simulink model "fixed_time_MASs"  (R2023b)
settings: Solver=FixedStepAuto  StartTime=0.0  StopTime=20  FixedStep=0.0001  RelTol=1e-3
(part 1 of 2)
settings Model: Creator=hxk  LastModifiedBy=hxk

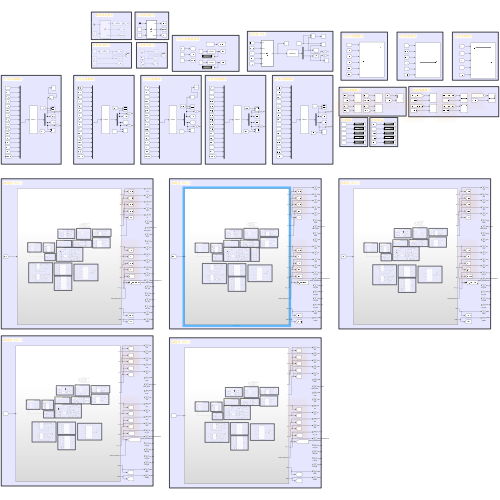
[thumbnail: Simulink's stored preview of the top-level diagram]
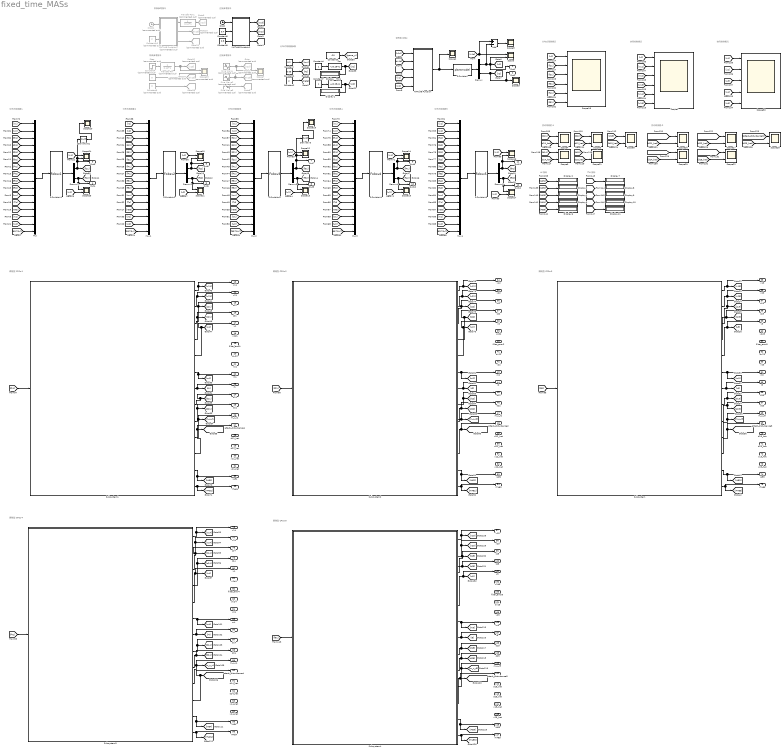
== system fixed_time_MASs ==
  note: 分布式观测情况
  note: 分布式观测器3
  note: 领导型 CPSs
  note: 分布式观测器1
  note: 分布式观测器2
  note: 分布式观测器参数
  note: 正弦参考指令
  note: 分布式观测器5
  note: 分布式观测器4
  note: 阶跃参考指令
  note: 协同控制情况
  note: 正弦参考指令
  note: 阶跃参考指令
  note: 跟随型 CPSs-3
  note: 跟随型 CPSs-1
  note: 跟随型 CPSs-2
  note: 跟随型 CPSs-4
  note: 跟随型 CPSs-5
  note: 扰动观测器-1
  note: 扰动观测器-2
  note: 协同控制情况
  note: IAE指标
  note: ITAE指标
  Add : Sum  Inputs=+-
  Clock : Clock
  Clock1 : Clock  Commented=on
  Constant : Constant  Value=0.2
  Constant1 : Constant  Value=0.05
  Constant10 : Constant  Commented=on  Value=2
  Constant2 : Constant  Value=2
  Constant3 : Constant  Value=-20
  Constant4 : Constant
  Constant5 : Constant  Commented=on  Value=0
  Constant6 : Constant  Commented=on  Value=0
  Constant7 : Constant
  Constant8 : Constant  Value=0.4
  Constant9 : Constant  Value=0.8
  Demux{,1..5} (6 alike) : Demux  Outputs=2
  Derivative : Derivative
  Derivative1 : Derivative
  Display{,1..11} (12 alike) : Display
  Fcn : Fcn  Expr=-u/0.2841
  Fcn1 : Fcn  Expr=-u/0.2841
  Goto : Goto  Commented=on  GotoTag=x1d
  Goto1 : Goto  Commented=on  GotoTag=dx1d
  Goto10 : Goto  Commented=on  GotoTag=dx1d
  Goto20 : Goto  Commented=on  GotoTag=ddx1d
  Goto56 : Goto  Commented=on  GotoTag=x1d
  Goto57 : Goto  Commented=on  GotoTag=dx1d
  Goto58 : Goto  Commented=on  GotoTag=ddx1d
  Goto8 : Goto  Commented=on  GotoTag=ddx1d
  Goto9 : Goto  Commented=on  GotoTag=x1d
  MATLAB Function : MATLAB Function  TreatAsAtomicUnit=on
  MATLAB Function1 : MATLAB Function  TreatAsAtomicUnit=on
  MATLAB Function2 : MATLAB Function  Commented=on  TreatAsAtomicUnit=on
  Mux{,1..4} (5 alike) : Mux  Inputs=16
  S-Function : S-Function  FunctionName=plantmodel  SFunctionDeploymentMode=off  EnableBusSupport=off
  S-Function1 : S-Function  FunctionName=Fobsv1  SFunctionDeploymentMode=off  EnableBusSupport=off
  S-Function2 : S-Function  FunctionName=Fobsv2  SFunctionDeploymentMode=off  EnableBusSupport=off
  S-Function3 : S-Function  FunctionName=Fobsv3  SFunctionDeploymentMode=off  EnableBusSupport=off
  S-Function4 : S-Function  FunctionName=Fobsv4  SFunctionDeploymentMode=off  EnableBusSupport=off
  S-Function5 : S-Function  FunctionName=Fobsv5  SFunctionDeploymentMode=off  EnableBusSupport=off
  Scope{,4,6,8..17,21..22,24..29} (21 alike) : Scope  NumInputPorts=2
  Scope1 : Scope  NumInputPorts=6
  Scope18 : Scope  NumInputPorts=6
  Scope{2..3,5,19..20} (5 alike) : Scope
  Scope23 : Scope  Commented=on  NumInputPorts=2
  Scope30 : Scope  NumInputPorts=5
  Scope7 : Scope  Commented=on  NumInputPorts=2
  Sine Wave : Sin  Commented=on  Amplitude=2  SampleTime=0
  Sine Wave2 : Sin  Commented=on  Amplitude=2  Phase=pi/2  SampleTime=0
  Sine Wave3 : Sin  Commented=on  Amplitude=-2  SampleTime=0
  Step : Step  Commented=on  Time=10  After=5  SampleTime=0
  Subsystem : Subsystem
  Subsystem1 : Subsystem
  Subsystem2 : Subsystem
  Subsystem3 : Subsystem
  Subsystem4 : Subsystem
  Transfer Fcn : TransferFcn  Commented=on  Denominator=[0.1 1]
  Transfer Fcn1 : TransferFcn  Commented=on  Denominator=[0.1 1]
  Out1 : Outport  SignalName=x1
  Out2 : Outport  Port=2  SignalName=x2
  Out3 : Outport  Port=3  SignalName=f11
  Out4 : Outport  Port=4  SignalName=f12
  Out5 : Outport  Port=5  SignalName=f21
  Out6 : Outport  Port=6  SignalName=f22
  Out7 : Outport  Port=7  SignalName=f31
  Out8 : Outport  Port=8  SignalName=f32
  Out9 : Outport  Port=9  SignalName=f41
  Out10 : Outport  Port=10  SignalName=f42
  Out11 : Outport  Port=11  SignalName=f51
  Out12 : Outport  Port=12  SignalName=f52
  x11 : Outport  Port=13  SignalName=x11
  x21 : Outport  Port=14  SignalName=x21
  z11 : Outport  Port=15  SignalName=z11
  z21 : Outport  Port=16  SignalName=z21
  u1 : Outport  Port=17  SignalName=u1
  x2d1 : Outport  Port=18  SignalName=x2d1
  filter_error1 : Outport  Port=19  SignalName=filter_error1
  dv21 : Outport  Port=20  SignalName=dv21
  v21 : Outport  Port=21  SignalName=v21
  m1 : Outport  Port=22  SignalName=m1
  r1 : Outport  Port=23  SignalName=r1
  d11 : Outport  Port=24  SignalName=d11
  d21 : Outport  Port=25  SignalName=d21
  m_u_r1 : Outport  Port=26  SignalName=m_u_r1
  attack_disturbance1 : Outport  Port=27  SignalName=attack_disturbance1
  d11_hat : Outport  Port=28  SignalName=d11_hat
  d21_hat : Outport  Port=29  SignalName=d21_hat
  x11_hat : Outport  Port=30  SignalName=x11_hat
  x21_hat : Outport  Port=31  SignalName=x21_hat
  IAE1 : Outport  Port=32  SignalName=IAE1
  ITAE1 : Outport  Port=33  SignalName=ITAE1
  x12 : Outport  Port=34  SignalName=x12
  x22 : Outport  Port=35  SignalName=x22
  z12 : Outport  Port=36  SignalName=z12
  z22 : Outport  Port=37  SignalName=z22
  u2 : Outport  Port=38  SignalName=u2
  x2d2 : Outport  Port=39  SignalName=x2d2
  filter_error2 : Outport  Port=40  SignalName=filter_error2
  dv22 : Outport  Port=41  SignalName=dv22
  v22 : Outport  Port=42  SignalName=v22
  m2 : Outport  Port=43  SignalName=m2
  r2 : Outport  Port=44  SignalName=r2
  d12 : Outport  Port=45  SignalName=d12
  d22 : Outport  Port=46  SignalName=d22
  m_u_r2 : Outport  Port=47  SignalName=m_u_r2
  attack_disturbance2 : Outport  Port=48  SignalName=attack_disturbance2
  d12_hat : Outport  Port=49  SignalName=d12_hat
  d22_hat : Outport  Port=50  SignalName=d22_hat
  x12_hat : Outport  Port=51  SignalName=x12_hat
  x22_hat : Outport  Port=52  SignalName=x22_hat
  IAE2 : Outport  Port=53  SignalName=IAE2
  ITAE2 : Outport  Port=54  SignalName=ITAE2
  x13 : Outport  Port=55  SignalName=x13
  x23 : Outport  Port=56  SignalName=x23
  z13 : Outport  Port=57  SignalName=z13
  z23 : Outport  Port=58  SignalName=z23
  u3 : Outport  Port=59  SignalName=u3
  x2d3 : Outport  Port=60  SignalName=x2d3
  filter_error3 : Outport  Port=61  SignalName=filter_error3
  dv23 : Outport  Port=62  SignalName=dv23
  v23 : Outport  Port=63  SignalName=v23
  m3 : Outport  Port=64  SignalName=m3
  r3 : Outport  Port=65  SignalName=r3
  d13 : Outport  Port=66  SignalName=d13
  d23 : Outport  Port=67  SignalName=d23
  m_u_r3 : Outport  Port=68  SignalName=m_u_r3
  attack_disturbance3 : Outport  Port=69  SignalName=attack_disturbance3
  d13_hat : Outport  Port=70  SignalName=d13_hat
  d23_hat : Outport  Port=71  SignalName=d23_hat
  x13_hat : Outport  Port=72  SignalName=x13_hat
  x23_hat : Outport  Port=73  SignalName=x23_hat
  IAE3 : Outport  Port=74  SignalName=IAE3
  ITAE3 : Outport  Port=75  SignalName=ITAE3
  x14 : Outport  Port=76  SignalName=x14
  x24 : Outport  Port=77  SignalName=x24
  z14 : Outport  Port=78  SignalName=z14
  z24 : Outport  Port=79  SignalName=z24
  u4 : Outport  Port=80  SignalName=u4
  x2d4 : Outport  Port=81  SignalName=x2d4
  filter_error4 : Outport  Port=82  SignalName=filter_error4
  dv24 : Outport  Port=83  SignalName=dv24
  v24 : Outport  Port=84  SignalName=v24
  m4 : Outport  Port=85  SignalName=m4
  r4 : Outport  Port=86  SignalName=r4
  d14 : Outport  Port=87  SignalName=d14
  d24 : Outport  Port=88  SignalName=d24
  m_u_r4 : Outport  Port=89  SignalName=m_u_r4
  attack_disturbance4 : Outport  Port=90  SignalName=attack_disturbance4
  d14_hat : Outport  Port=91  SignalName=d14_hat
  d24_hat : Outport  Port=92  SignalName=d24_hat
  x14_hat : Outport  Port=93  SignalName=x14_hat
  x24_hat : Outport  Port=94  SignalName=x24_hat
  IAE4 : Outport  Port=95  SignalName=IAE4
  ITAE4 : Outport  Port=96  SignalName=ITAE4
  x15 : Outport  Port=97  SignalName=x15
  x25 : Outport  Port=98  SignalName=x25
  z15 : Outport  Port=99  SignalName=z15
  z25 : Outport  Port=100  SignalName=z25
  u5 : Outport  Port=101  SignalName=u5
  x2d5 : Outport  Port=102  SignalName=x2d5
  filter_error5 : Outport  Port=103  SignalName=filter_error5
  dv25 : Outport  Port=104  SignalName=dv25
  v25 : Outport  Port=105  SignalName=v25
  m5 : Outport  Port=106  SignalName=m5
  r5 : Outport  Port=107  SignalName=r5
  d15 : Outport  Port=108  SignalName=d15
  d25 : Outport  Port=109  SignalName=d25
  m_u_r5 : Outport  Port=110  SignalName=m_u_r5
  attack_disturbance5 : Outport  Port=111  SignalName=attack_disturbance5
  d15_hat : Outport  Port=112  SignalName=d15_hat
  d25_hat : Outport  Port=113  SignalName=d25_hat
  x15_hat : Outport  Port=114  SignalName=x15_hat
  x25_hat : Outport  Port=115  SignalName=x25_hat
  IAE5 : Outport  Port=116  SignalName=IAE5
  ITAE5 : Outport  Port=117  SignalName=ITAE5
  wires:
  [Tc] -> Mux2/12
  Derivative1/1 -> Scope20/1
  Constant3/1 -> [gama_n]
  Demux5/2 -> Out12/1, Scope17/1, [f52]
  [f32] -> Mux3/8
  [mu] -> Mux/11
  [f32] -> Mux1/6
  [x1] -> MATLAB Function/4(x1)
  S-Function/1 -> Demux/1
  [f51] -> Scope18/6
  Derivative/1 -> Scope19/1
  Mux4/1 -> S-Function5/1
  Sine Wave3/1 -> Goto8/1
  [f32] -> Mux/6
  [x1] -> Mux2/1
  Sine Wave2/1 -> Scope7/2, Goto1/1
  Constant1/1 -> [Tc]
  [x1] -> Scope10/1
  [f52] -> Mux3/10
  [f22] -> Mux3/6
  Demux3/1 -> Out7/1, Derivative/1, Scope12/2, [f31]
  [f51] -> Mux3/9
  [Tc] -> Mux1/12
  [f22] -> Mux2/6
  [f41] -> Scope18/5
  [x1] -> Mux4/1
  [x2] -> Scope13/2
  Mux2/1 -> S-Function3/1
  [x1] -> Mux/1
  [f12] -> Mux1/4
  S-Function4/1 -> Demux4/1
  [f51] -> Mux2/9
  [f51] -> Mux/9
  Transfer Fcn/1 -> Goto56/1, Scope23/1
  [x1] -> Scope14/1
  [Tc] -> Mux4/12
  Demux/2 -> Scope3/1, Out2/1, [x2]
  [mu] -> Mux1/11
  Constant/1 -> [mu]
  [mu] -> Mux4/11
  S-Function1/1 -> Demux1/1
  [f12] -> Mux2/4
  Demux/1 -> Add/2, Out1/1, Scope/2, [x1]
  [x2] -> Mux4/2
  [f22] -> Mux/4
  [f11] -> Mux2/3
  [f31] -> Mux/5
  [neta] -> Mux/13
  Add/1 -> Scope5/1
  [mu] -> Mux3/11
  [f31] -> Mux1/5
  [x1] -> Mux1/1
  [x1] -> Scope24/1
  [f42] -> Mux1/8
  MATLAB Function/1(u0) -> Scope2/1, S-Function/1
  [f42] -> Mux/8
  Fcn/1 -> Display/1, [w1]
  [f51] -> Mux1/9
  Demux1/2 -> Scope25/1, Out4/1, [f12]
  Mux1/1 -> S-Function2/1
  [f21] -> Mux/3
  [f41] -> Mux/7
  [f12] -> Mux3/4
  Demux4/1 -> Out9/1, Scope14/2, [f41]
  [f21] -> Mux2/5
  Constant4/1 -> Fcn/1
  [x2] -> Scope17/2
  Constant2/1 -> [neta]
  [f31] -> Mux4/7
  [x2] -> Mux/2
  [x2] -> Mux2/2
  [x1d] -> MATLAB Function/1(x1d)
  Mux3/1 -> S-Function4/1
  Demux2/2 -> [f22], Scope11/1, Out6/1
  Demux5/1 -> Out11/1, Scope16/2, [f51]
  [f22] -> Mux4/6
  [x2] -> Scope15/2
  [f32] -> Mux4/8
  [x1] -> Scope12/1
  [f41] -> Mux4/9
  [dx1d] -> MATLAB Function/2(dx1d)
  [f41] -> Mux1/7
  S-Function2/1 -> Demux2/1
  [f12] -> Mux4/4
  [f41] -> Mux2/7
  Demux3/2 -> Out8/1, Scope13/1, [f32]
  [x1] -> Scope18/1
  Constant6/1 -> Goto57/1, Scope23/2
  [f21] -> Scope18/3
  [x2] -> Scope25/2
  [ddx1d] -> MATLAB Function/3(ddx1d)
  [f11] -> Scope18/2
  Demux4/2 -> [f42], Out10/1, Scope15/1
  [f21] -> Mux4/5
  [f42] -> Mux2/8
  [f21] -> Mux3/5
  Mux/1 -> S-Function1/1
  [x1] -> Scope16/1
  [x2] -> MATLAB Function/5(x2)
  [x2] -> Mux1/2
  [f11] -> Mux4/3
  S-Function3/1 -> Demux3/1
  [f31] -> Scope18/4
  [f31] -> Mux3/7
  [w2] -> Mux/15
  [Tc] -> Mux3/12
  [mu] -> Mux2/11
  [f11] -> Mux3/3
  Constant5/1 -> Goto58/1
  [f52] -> Mux1/10
  Step/1 -> Transfer Fcn/1
  [f52] -> Mux2/10
  [f42] -> Mux4/10
  S-Function5/1 -> Demux5/1
  [x2] -> Mux3/2
  [x1d] -> Add/1, Scope/1
  [x2] -> Scope11/2
  Demux2/1 -> Out5/1, Scope10/2, [f21]
  Demux1/1 -> Derivative1/1, Scope24/2, Out3/1, [f11]
  [f11] -> Mux1/3
  [Tc] -> Mux/12
  [w1] -> Mux/14
  [x1] -> Mux3/1
  [f52] -> Mux/10
  Sine Wave/1 -> Scope7/1, Goto/1
  [x13] -> Scope1/4
  [x11] -> Scope1/2
  [x12] -> Scope1/3
  [x1] -> Scope1/1
  [x14] -> Scope1/5
  [x15] -> Scope1/6
  Clock/1 -> MATLAB Function1/1(t)
  Constant8/1 -> MATLAB Function1/2(a)
  Constant9/1 -> MATLAB Function1/3(b)
  MATLAB Function1/1(x1d) -> [x1d]
  MATLAB Function1/2(dx1d) -> [dx1d]
  MATLAB Function1/3(ddx1d) -> [ddx1d]
  MATLAB Function2/3(ddx1d) -> Goto20/1
  MATLAB Function2/2(dx1d) -> Goto10/1
  MATLAB Function2/1(x1d) -> Transfer Fcn1/1
  Clock1/1 -> MATLAB Function2/1(t)
  Transfer Fcn1/1 -> Goto9/1
  Constant10/1 -> MATLAB Function2/2(a)
  Constant7/1 -> Fcn1/1
  Fcn1/1 -> [w2], Display1/1
  [gama_n] -> Mux/16
  [gama_n] -> Mux1/16
  [w1] -> Mux1/14
  [w2] -> Mux1/15
  [neta] -> Mux1/13
  [neta] -> Mux2/13
  [w2] -> Mux2/15
  [w1] -> Mux2/14
  [gama_n] -> Mux2/16
  [gama_n] -> Mux3/16
  [w1] -> Mux3/14
  [w2] -> Mux3/15
  [neta] -> Mux3/13
  [neta] -> Mux4/13
  [w2] -> Mux4/15
  [w1] -> Mux4/14
  [gama_n] -> Mux4/16
  [f31] -> Subsystem/1(In1)
  Subsystem/1(x1) -> x13/1, [x13]
  Subsystem/2(x2) -> x23/1, [x23]
  Subsystem/3(z1) -> z13/1, [z13]
  Subsystem/4(z2) -> z23/1, [z23]
  Subsystem/5(u) -> u3/1, [u3]
  Subsystem/6(m) -> [m3], m3/1
  Subsystem/7(r) -> r3/1, [r3]
  Subsystem/8(d1) -> d13/1, [d13]
  Subsystem/9(d2) -> [d23], d23/1
  Subsystem/10(m_u_r) -> m_u_r3/1, [m_u_r3]
  Subsystem/11(attack_disturbance) -> attack_disturbance3/1, [attack_disturbance3]
  Subsystem/12(IAE) -> [IAE3], IAE3/1
  Subsystem/13(ITAE) -> [ITAE3], ITAE3/1
  Subsystem1/13(ITAE) -> [ITAE1], ITAE1/1
  Subsystem1/12(IAE) -> [IAE1], IAE1/1
  Subsystem1/11(attack_disturbance) -> attack_disturbance1/1, [attack_disturbance1]
  Subsystem1/10(m_u_r) -> m_u_r1/1, [m_u_r1]
  Subsystem1/9(d2) -> d21/1, [d21]
  Subsystem1/8(d1) -> d11/1, [d11]
  Subsystem1/7(r) -> r1/1, [r1]
  Subsystem1/6(m) -> [m1], m1/1
  Subsystem1/5(u) -> u1/1, [u1]
  Subsystem1/4(z2) -> z21/1, [z21]
  Subsystem1/3(z1) -> z11/1, [z11]
  Subsystem1/2(x2) -> x21/1, [x21]
  Subsystem1/1(x1) -> x11/1, [x11]
  [f11] -> Subsystem1/1(In1)
  [f21] -> Subsystem2/1(In1)
  Subsystem2/1(x1) -> x12/1, [x12]
  Subsystem2/2(x2) -> x22/1, [x22]
  Subsystem2/3(z1) -> z12/1, [z12]
  Subsystem2/4(z2) -> z22/1, [z22]
  Subsystem2/5(u) -> u2/1, [u2]
  Subsystem2/6(m) -> [m2], m2/1
  Subsystem2/7(r) -> r2/1, [r2]
  Subsystem2/8(d1) -> d12/1, [d12]
  Subsystem2/9(d2) -> d22/1, [d22]
  Subsystem2/10(m_u_r) -> m_u_r2/1, [m_u_r2]
  Subsystem2/11(attack_disturbance) -> [attack_disturbance2], attack_disturbance2/1
  Subsystem2/12(IAE) -> [IAE2], IAE2/1
  Subsystem2/13(ITAE) -> [ITAE2], ITAE2/1
  Subsystem3/13(ITAE) -> [ITAE4], ITAE4/1
  Subsystem3/12(IAE) -> [IAE4], IAE4/1
  Subsystem3/11(attack_disturbance) -> attack_disturbance4/1, [attack_disturbance4]
  Subsystem3/10(m_u_r) -> m_u_r4/1, [m_u_r4]
  Subsystem3/9(d2) -> d24/1, [d24]
  Subsystem3/8(d1) -> d14/1, [d14]
  Subsystem3/7(r) -> r4/1, [r4]
  Subsystem3/6(m) -> [m4], m4/1
  Subsystem3/5(u) -> u4/1, [u4]
  Subsystem3/4(z2) -> z24/1, [z24]
  Subsystem3/3(z1) -> z14/1, [z14]
  Subsystem3/2(x2) -> x24/1, [x24]
  Subsystem3/1(x1) -> x14/1, [x14]
  [f41] -> Subsystem3/1(In1)
  [f51] -> Subsystem4/1(In1)
  Subsystem4/1(x1) -> x15/1, [x15]
  Subsystem4/2(x2) -> x25/1, [x25]
  Subsystem4/3(z1) -> z15/1, [z15]
  Subsystem4/4(z2) -> z25/1, [z25]
  Subsystem4/5(u) -> u5/1, [u5]
  Subsystem4/6(m) -> [m5], m5/1
  Subsystem4/7(r) -> r5/1, [r5]
  Subsystem4/8(d1) -> d15/1, [d15]
  Subsystem4/9(d2) -> d25/1, [d25]
  Subsystem4/10(m_u_r) -> m_u_r5/1, [m_u_r5]
  Subsystem4/11(attack_disturbance) -> attack_disturbance5/1, [attack_disturbance5]
  Subsystem4/12(IAE) -> [IAE5], IAE5/1
  Subsystem4/13(ITAE) -> [ITAE5], ITAE5/1
  [d11] -> Scope4/1
  [d11_hat] -> Scope4/2
  [d12_hat] -> Scope6/2
  [d12] -> Scope6/1
  [d13] -> Scope8/1
  [d13_hat] -> Scope8/2
  [d15] -> Scope21/1
  [d15_hat] -> Scope21/2
  [d14_hat] -> Scope9/2
  [d14] -> Scope9/1
  [attack_disturbance4] -> Scope29/1
  [d24_hat] -> Scope29/2
  [d25_hat] -> Scope22/2
  [attack_disturbance5] -> Scope22/1
  [d23_hat] -> Scope28/2
  [attack_disturbance3] -> Scope28/1
  [attack_disturbance2] -> Scope27/1
  [d22_hat] -> Scope27/2
  [d21_hat] -> Scope26/2
  [attack_disturbance1] -> Scope26/1
  [u5] -> Scope30/5
  [u1] -> Scope30/1
  [u3] -> Scope30/3
  [u2] -> Scope30/2
  [u4] -> Scope30/4
  [IAE1] -> Display2/1
  [IAE2] -> Display3/1
  [IAE3] -> Display4/1
  [IAE4] -> Display5/1
  [IAE5] -> Display6/1
  [ITAE5] -> Display11/1
  [ITAE4] -> Display10/1
  [ITAE3] -> Display9/1
  [ITAE2] -> Display8/1
  [ITAE1] -> Display7/1

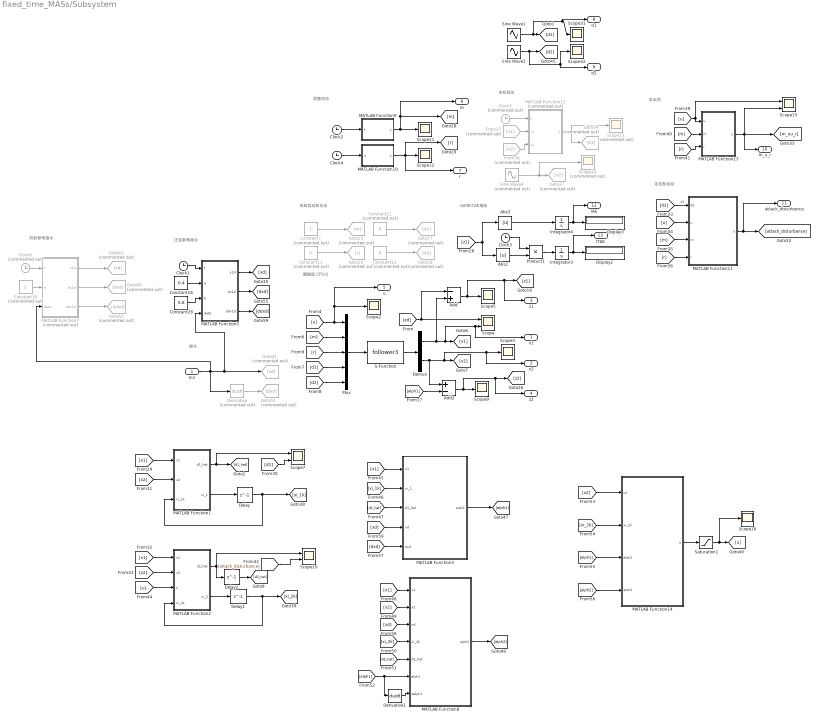
== system fixed_time_MASs/Subsystem ==
  note: 跟随型 CPSs1
  note: 未知扰动和攻击
  note: IAE和ITAE指标
  note: 恶意攻击
  note: 未知扰动
  note: 攻击和扰动
  note: 攻击项
  note: 正弦参考指令
  note: 阶跃参考指令
  note: 指令
  In1 : Inport
  Abs2 : Abs  SaturateOnIntegerOverflow=off
  Abs3 : Abs  SaturateOnIntegerOverflow=off
  Add : Sum  Inputs=-+
  Add2 : Sum  Inputs=+-
  Clock{1..4} (4 alike) : Clock
  Clock5 : Clock  Commented=on
  Clock6 : Clock  Commented=on
  Constant11 : Constant  Commented=on  Value=0
  Constant12 : Constant  Commented=on  Value=0
  Constant13 : Constant  Commented=on  Value=0
  Constant16 : Constant  Value=0.4
  Constant28 : Constant  Value=0.8
  Constant30 : Constant  Commented=on  Value=2
  Constant7 : Constant  Commented=on
  Delay : Delay  DelayLength=1  InitialCondition=0
  Delay1 : Delay  DelayLength=1  InitialCondition=0
  Delay2 : Delay  DelayLength=1  InitialCondition=0
  Demux : Demux  Outputs=2
  Derivative : Derivative  Commented=on
  Derivative1 : Derivative
  Display2 : Display
  Display3 : Display
  From37 : From  Commented=on  GotoTag=x1
  From38 : From  Commented=on  GotoTag=x2
  Goto15 : Goto  Commented=on  GotoTag=m
  Goto16 : Goto  Commented=on  GotoTag=r
  Goto17 : Goto  Commented=on  GotoTag=d1
  Goto18 : Goto  Commented=on  GotoTag=d2
  Goto34 : Goto  Commented=on  GotoTag=d1
  Goto37 : Goto  Commented=on  GotoTag=d2
  Goto41 : Goto  Commented=on  GotoTag=xd
  Goto53 : Goto  Commented=on  GotoTag=dxd
  Goto60 : Goto  Commented=on  GotoTag=dxd
  Goto62 : Goto  Commented=on  GotoTag=ddxd
  Goto63 : Goto  Commented=on  GotoTag=xd
  Integrator3 : Integrator
  Integrator4 : Integrator
  MATLAB Function1 : MATLAB Function  TreatAsAtomicUnit=on
  MATLAB Function10 : MATLAB Function  TreatAsAtomicUnit=on
  MATLAB Function11 : MATLAB Function  TreatAsAtomicUnit=on
  MATLAB Function12 : MATLAB Function  Commented=on  TreatAsAtomicUnit=on
  MATLAB Function13 : MATLAB Function  TreatAsAtomicUnit=on
  MATLAB Function14 : MATLAB Function  TreatAsAtomicUnit=on
  MATLAB Function2 : MATLAB Function  TreatAsAtomicUnit=on
  MATLAB Function3 : MATLAB Function  TreatAsAtomicUnit=on
  MATLAB Function5 : MATLAB Function  TreatAsAtomicUnit=on
  MATLAB Function7 : MATLAB Function  Commented=on  TreatAsAtomicUnit=on
  MATLAB Function8 : MATLAB Function  TreatAsAtomicUnit=on
  MATLAB Function9 : MATLAB Function  TreatAsAtomicUnit=on
  Mux : Mux  Inputs=5
  Product1 : Product
  S-Function : S-Function  FunctionName=follower3  SFunctionDeploymentMode=off  EnableBusSupport=off
  Saturation1 : Saturate  UpperLimit=1000  LowerLimit=-1000
  Scope{,7,10,15} (4 alike) : Scope  NumInputPorts=2
  Scope{2..3,5,9,11..12,16,31..32} (9 alike) : Scope
  Scope13 : Scope  Commented=on
  Scope14 : Scope  Commented=on
  Sine Wave1 : Sin  Amplitude=0.8  Phase=pi/2  SampleTime=0
  Sine Wave2 : Sin  Amplitude=0.8*0.8  SampleTime=0
  Sine Wave4 : Sin  Commented=on  Amplitude=3  Phase=pi/2  SampleTime=0
  x1 : Outport
  x2 : Outport  Port=2
  z1 : Outport  Port=3
  z2 : Outport  Port=4
  u : Outport  Port=5
  m : Outport  Port=6
  r : Outport  Port=7
  d1 : Outport  Port=8
  d2 : Outport  Port=9
  m_u_r : Outport  Port=10
  attack_disturbance : Outport  Port=11
  IAE : Outport  Port=12
  ITAE : Outport  Port=13
  wires:
  [xd] -> Add/1, Scope/1
  Abs3/1 -> Integrator4/1
  [r] -> MATLAB Function13/3(r)
  Demux/2 -> Add2/1, Scope3/1, x2/1, [x2]
  Constant11/1 -> Goto16/1
  Constant13/1 -> Goto18/1
  MATLAB Function13/1(y) -> m_u_r/1, [m_uu_r], Scope15/2
  Demux/1 -> Add/2, x1/1, Scope/2, [x1]
  Add/1 -> z1/1, [z1], Scope5/1
  [u] -> u/1, Scope2/1, Mux/1
  Product1/1 -> Integrator3/1
  S-Function/1 -> Demux/1
  [d1] -> Mux/4
  Clock3/1 -> Product1/1
  [d2] -> MATLAB Function11/1(d2)  "d1"
  Integrator4/1 -> IAE/1, Display3/1
  [m] -> Mux/2
  Abs2/1 -> Product1/2
  Integrator3/1 -> ITAE/1, Display2/1
  [r] -> MATLAB Function11/4(r)
  [z1] -> Abs2/1, Abs3/1
  Constant7/1 -> Goto15/1
  [r] -> Mux/3
  [d2] -> Mux/5
  Constant12/1 -> Goto17/1
  Mux/1 -> S-Function/1
  MATLAB Function10/1(y) -> r/1, [r], Scope12/1
  Add2/1 -> z2/1, [z2], Scope9/1
  MATLAB Function12/1(y) -> Goto34/1, Scope13/1
  Clock4/1 -> MATLAB Function10/1(u)
  Clock2/1 -> MATLAB Function9/1(t)
  MATLAB Function9/1(y) -> m/1, [m], Scope11/1
  [alph1] -> Add2/2
  [u] -> MATLAB Function11/2(u)
  [m] -> MATLAB Function11/3(m)
  MATLAB Function11/1(y) -> attack_disturbance/1, [attack_disturbance]
  [u] -> Scope15/1, MATLAB Function13/1(u)
  Sine Wave4/1 -> Scope14/1, Goto37/1
  From38/1 -> MATLAB Function12/3(x2)
  From37/1 -> MATLAB Function12/2(x1)
  Clock5/1 -> MATLAB Function12/1(t)
  [m] -> MATLAB Function13/2(m)
  Sine Wave1/1 -> d1/1, Scope31/1, [d1]
  Sine Wave2/1 -> Scope32/1, d2/1, [d2]
  MATLAB Function5/1(x1d) -> [xd]
  Constant16/1 -> MATLAB Function5/2(a)
  Constant28/1 -> MATLAB Function5/3(b)
  MATLAB Function7/3(ddx1d) -> Goto62/1
  Constant30/1 -> MATLAB Function7/2(a)
  MATLAB Function7/2(dx1d) -> Goto60/1
  In1/1 -> MATLAB Function7/3(data), MATLAB Function5/4(data), Goto41/1, Derivative/1
  Clock1/1 -> MATLAB Function5/1(t)
  Clock6/1 -> MATLAB Function7/1(t)
  Derivative/1 -> Goto53/1
  MATLAB Function5/3(ddx1d) -> [ddxd]
  MATLAB Function5/2(dx1d) -> [dxd]
  MATLAB Function7/1(x1d) -> Goto63/1
  Derivative1/1 -> MATLAB Function8/7(dalph1)
  [x2] -> MATLAB Function8/2(x2)
  [alph1] -> MATLAB Function8/6(alph1), Derivative1/1
  Saturation1/1 -> Scope16/1, [u]
  [x1] -> MATLAB Function8/1(x1)
  [x2] -> MATLAB Function1/2(x2)
  [xi_2k] -> MATLAB Function8/4(xi_2k)
  [xd] -> MATLAB Function3/4(xd)
  [u] -> MATLAB Function2/3(u)
  MATLAB Function3/1(alph1) -> [alph1]
  [alph1] -> MATLAB Function14/3(alph1)
  Delay1/1 -> [xi_2k], MATLAB Function2/4(xi_2k)
  Delay/1 -> [xi_1k], MATLAB Function1/3(xi_1k)
  MATLAB Function8/1(alph2) -> [alph2]
  Delay2/1 -> [d2_hat]
  [x2] -> MATLAB Function14/1(x2)
  [d2_hat] -> MATLAB Function8/5(d2_hat)
  [dxd] -> MATLAB Function3/5(dxd)
  MATLAB Function2/2(xi_2) -> Delay1/1
  [x1] -> MATLAB Function2/1(x1)
  MATLAB Function2/1(d2_hat) -> Delay2/1, Scope10/1
  [xd] -> MATLAB Function8/3(xd)
  [alph2] -> MATLAB Function14/4(alph2)
  [x2] -> MATLAB Function2/2(x2)
  [xi_1k] -> MATLAB Function3/2(xi_1)
  [x1] -> MATLAB Function3/1(x1)
  [d1] -> Scope7/2
  [xi_2k] -> MATLAB Function14/2(xi_2k)
  [attack_disturbance] -> Scope10/2
  [d1_hat] -> MATLAB Function3/3(d1_hat)
  MATLAB Function1/2(xi_1) -> Delay/1
  MATLAB Function14/1(u) -> Saturation1/1
  MATLAB Function1/1(d1_hat) -> Scope7/1, [d1_hat]
  [x1] -> MATLAB Function1/1(x1)

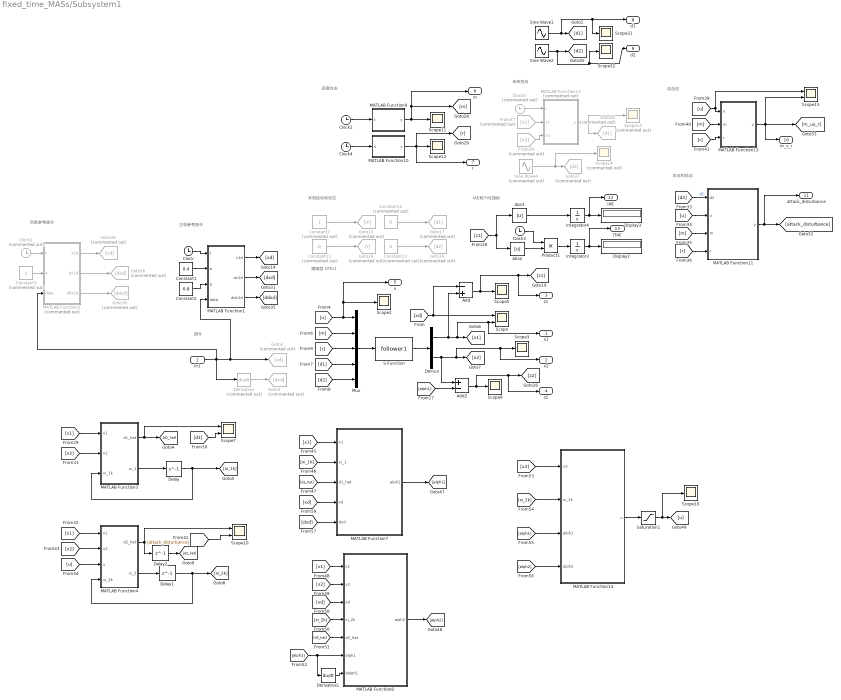
== system fixed_time_MASs/Subsystem1 ==
  note: 指令
  note: 攻击项
  note: 攻击和扰动
  note: 未知扰动
  note: 恶意攻击
  note: IAE和ITAE指标
  note: 未知扰动和攻击
  note: 跟随型 CPSs1
  note: 正弦参考指令
  note: 阶跃参考指令
  In1 : Inport
  Abs2 : Abs  SaturateOnIntegerOverflow=off
  Abs3 : Abs  SaturateOnIntegerOverflow=off
  Add : Sum  Inputs=-+
  Add2 : Sum  Inputs=+-
  Clock{,2..4} (4 alike) : Clock
  Clock1 : Clock  Commented=on
  Clock5 : Clock  Commented=on
  Constant1 : Constant  Value=0.4
  Constant11 : Constant  Commented=on  Value=0
  Constant12 : Constant  Commented=on  Value=0
  Constant13 : Constant  Commented=on  Value=0
  Constant2 : Constant  Value=0.8
  Constant3 : Constant  Commented=on  Value=2
  Constant7 : Constant  Commented=on
  Delay : Delay  DelayLength=1  InitialCondition=0
  Delay1 : Delay  DelayLength=1  InitialCondition=0
  Delay2 : Delay  DelayLength=1  InitialCondition=0
  Demux : Demux  Outputs=2
  Derivative : Derivative  Commented=on
  Derivative1 : Derivative
  Display2 : Display
  Display3 : Display
  From37 : From  Commented=on  GotoTag=x1
  From38 : From  Commented=on  GotoTag=x2
  Goto15 : Goto  Commented=on  GotoTag=m
  Goto16 : Goto  Commented=on  GotoTag=r
  Goto17 : Goto  Commented=on  GotoTag=d1
  Goto18 : Goto  Commented=on  GotoTag=d2
  Goto2 : Goto  Commented=on  GotoTag=xd
  Goto3 : Goto  Commented=on  GotoTag=dxd
  Goto34 : Goto  Commented=on  GotoTag=d1
  Goto36 : Goto  Commented=on  GotoTag=dxd
  Goto37 : Goto  Commented=on  GotoTag=d2
  Goto38 : Goto  Commented=on  GotoTag=ddxd
  Goto39 : Goto  Commented=on  GotoTag=xd
  Integrator3 : Integrator
  Integrator4 : Integrator
  MATLAB Function1 : MATLAB Function  TreatAsAtomicUnit=on
  MATLAB Function10 : MATLAB Function  TreatAsAtomicUnit=on
  MATLAB Function11 : MATLAB Function  TreatAsAtomicUnit=on
  MATLAB Function12 : MATLAB Function  Commented=on  TreatAsAtomicUnit=on
  MATLAB Function13 : MATLAB Function  TreatAsAtomicUnit=on
  MATLAB Function14 : MATLAB Function  TreatAsAtomicUnit=on
  MATLAB Function2 : MATLAB Function  Commented=on  TreatAsAtomicUnit=on
  MATLAB Function3 : MATLAB Function  TreatAsAtomicUnit=on
  MATLAB Function4 : MATLAB Function  TreatAsAtomicUnit=on
  MATLAB Function7 : MATLAB Function  TreatAsAtomicUnit=on
  MATLAB Function8 : MATLAB Function  TreatAsAtomicUnit=on
  MATLAB Function9 : MATLAB Function  TreatAsAtomicUnit=on
  Mux : Mux  Inputs=5
  Product1 : Product
  S-Function : S-Function  FunctionName=follower1  SFunctionDeploymentMode=off  EnableBusSupport=off
  Saturation1 : Saturate  UpperLimit=1000  LowerLimit=-1000
  Scope{,7,10,15} (4 alike) : Scope  NumInputPorts=2
  Scope{2..3,5,9,11..12,16,31..32} (9 alike) : Scope
  Scope13 : Scope  Commented=on
  Scope14 : Scope  Commented=on
  Sine Wave1 : Sin  Amplitude=0.2  Phase=pi/2  SampleTime=0
  Sine Wave2 : Sin  Amplitude=0.8*0.2  SampleTime=0
  Sine Wave4 : Sin  Commented=on  Amplitude=3  Phase=pi/2  SampleTime=0
  x1 : Outport
  x2 : Outport  Port=2
  z1 : Outport  Port=3
  z2 : Outport  Port=4
  u : Outport  Port=5
  m : Outport  Port=6
  r : Outport  Port=7
  d1 : Outport  Port=8
  d2 : Outport  Port=9
  m_u_r : Outport  Port=10
  attack_disturbance : Outport  Port=11
  IAE : Outport  Port=12
  ITAE : Outport  Port=13
  wires:
  [m] -> MATLAB Function13/2(m)
  Clock5/1 -> MATLAB Function12/1(t)
  From37/1 -> MATLAB Function12/2(x1)
  From38/1 -> MATLAB Function12/3(x2)
  Sine Wave4/1 -> Goto37/1, Scope14/1
  [u] -> MATLAB Function13/1(u), Scope15/1
  MATLAB Function11/1(y) -> [attack_disturbance], attack_disturbance/1
  [m] -> MATLAB Function11/3(m)
  [u] -> MATLAB Function11/2(u)
  [alph1] -> Add2/2
  MATLAB Function9/1(y) -> Scope11/1, [m], m/1
  Clock2/1 -> MATLAB Function9/1(t)
  Clock4/1 -> MATLAB Function10/1(u)
  MATLAB Function12/1(y) -> Scope13/1, Goto34/1
  Add2/1 -> Scope9/1, [z2], z2/1
  MATLAB Function10/1(y) -> Scope12/1, [r], r/1
  Mux/1 -> S-Function/1
  Constant12/1 -> Goto17/1
  [d2] -> Mux/5
  [r] -> Mux/3
  Constant7/1 -> Goto15/1
  [z1] -> Abs3/1, Abs2/1
  [r] -> MATLAB Function11/4(r)
  Integrator3/1 -> Display2/1, ITAE/1
  Derivative/1 -> Goto3/1
  Abs2/1 -> Product1/2
  [m] -> Mux/2
  Integrator4/1 -> Display3/1, IAE/1
  [d2] -> MATLAB Function11/1(d2)  "d1"
  Clock3/1 -> Product1/1
  [d1] -> Mux/4
  S-Function/1 -> Demux/1
  Product1/1 -> Integrator3/1
  [u] -> Mux/1, Scope2/1, u/1
  Add/1 -> Scope5/1, [z1], z1/1
  Demux/1 -> [x1], Scope/2, x1/1, Add/2
  MATLAB Function13/1(y) -> Scope15/2, [m_uu_r], m_u_r/1
  Constant13/1 -> Goto18/1
  Constant11/1 -> Goto16/1
  Demux/2 -> [x2], x2/1, Scope3/1, Add2/1
  [r] -> MATLAB Function13/3(r)
  Abs3/1 -> Integrator4/1
  [xd] -> Scope/1, Add/1
  In1/1 -> MATLAB Function2/3(data), MATLAB Function1/4(data), Goto2/1, Derivative/1
  Sine Wave1/1 -> d1/1, Scope31/1, [d1]
  Sine Wave2/1 -> d2/1, Scope32/1, [d2]
  Constant2/1 -> MATLAB Function1/3(b)
  Clock/1 -> MATLAB Function1/1(t)
  Constant1/1 -> MATLAB Function1/2(a)
  MATLAB Function1/2(dx1d) -> [dxd]
  MATLAB Function1/3(ddx1d) -> [ddxd]
  MATLAB Function1/1(x1d) -> [xd]
  Clock1/1 -> MATLAB Function2/1(t)
  Constant3/1 -> MATLAB Function2/2(a)
  MATLAB Function2/2(dx1d) -> Goto36/1
  MATLAB Function2/3(ddx1d) -> Goto38/1
  MATLAB Function2/1(x1d) -> Goto39/1
  Derivative1/1 -> MATLAB Function8/7(dalph1)
  [x2] -> MATLAB Function8/2(x2)
  [alph1] -> MATLAB Function8/6(alph1), Derivative1/1
  Saturation1/1 -> Scope16/1, [u]
  [x1] -> MATLAB Function8/1(x1)
  [x2] -> MATLAB Function3/2(x2)
  [xi_2k] -> MATLAB Function8/4(xi_2k)
  [xd] -> MATLAB Function7/4(xd)
  [u] -> MATLAB Function4/3(u)
  MATLAB Function7/1(alph1) -> [alph1]
  [alph1] -> MATLAB Function14/3(alph1)
  Delay1/1 -> [xi_2k], MATLAB Function4/4(xi_2k)
  Delay/1 -> [xi_1k], MATLAB Function3/3(xi_1k)
  MATLAB Function8/1(alph2) -> [alph2]
  Delay2/1 -> [d2_hat]
  [x2] -> MATLAB Function14/1(x2)
  [d2_hat] -> MATLAB Function8/5(d2_hat)
  [dxd] -> MATLAB Function7/5(dxd)
  MATLAB Function4/2(xi_2) -> Delay1/1
  [x1] -> MATLAB Function4/1(x1)
  MATLAB Function4/1(d2_hat) -> Delay2/1, Scope10/1
  [xd] -> MATLAB Function8/3(xd)
  [alph2] -> MATLAB Function14/4(alph2)
  [x2] -> MATLAB Function4/2(x2)
  [xi_1k] -> MATLAB Function7/2(xi_1)
  [x1] -> MATLAB Function7/1(x1)
  [d1] -> Scope7/2
  [xi_2k] -> MATLAB Function14/2(xi_2k)
  [attack_disturbance] -> Scope10/2
  [d1_hat] -> MATLAB Function7/3(d1_hat)
  MATLAB Function3/2(xi_1) -> Delay/1
  MATLAB Function14/1(u) -> Saturation1/1
  MATLAB Function3/1(d1_hat) -> Scope7/1, [d1_hat]
  [x1] -> MATLAB Function3/1(x1)

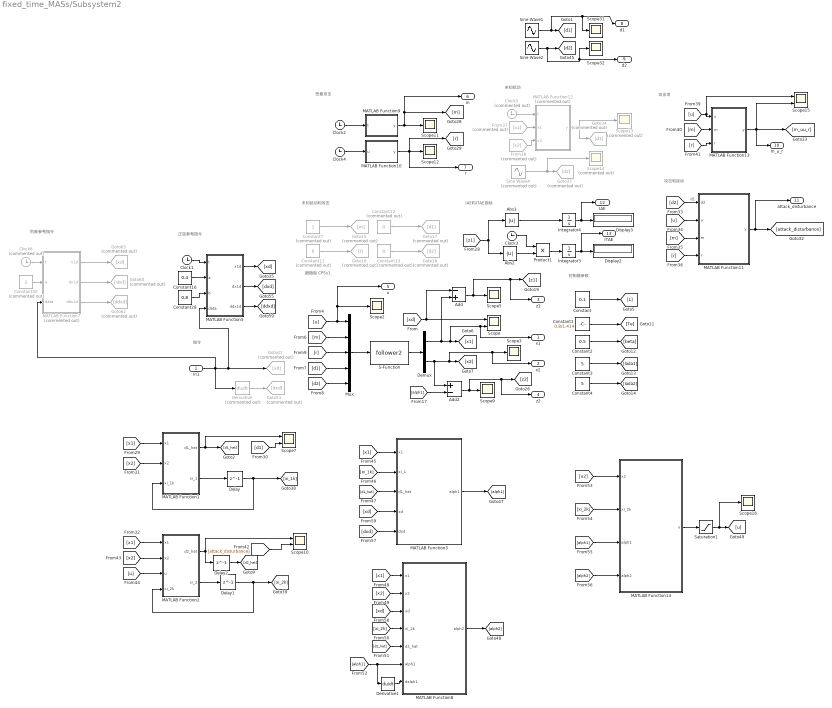
== system fixed_time_MASs/Subsystem2 ==
  note: 跟随型 CPSs1
  note: 控制器参数
  note: 未知扰动和攻击
  note: IAE和ITAE指标
  note: 恶意攻击
  note: 未知扰动
  note: 攻击和扰动
  note: 攻击项
  note: 正弦参考指令
  note: 阶跃参考指令
  note: 指令
  In1 : Inport
  Abs2 : Abs  SaturateOnIntegerOverflow=off
  Abs3 : Abs  SaturateOnIntegerOverflow=off
  Add : Sum  Inputs=-+
  Add2 : Sum  Inputs=+-
  Clock{1..4} (4 alike) : Clock
  Clock5 : Clock  Commented=on
  Clock6 : Clock  Commented=on
  Constant : Constant  Value=0.1
  Constant1 : Constant  Value=0.8/1.414
  Constant11 : Constant  Commented=on  Value=0
  Constant12 : Constant  Commented=on  Value=0
  Constant13 : Constant  Commented=on  Value=0
  Constant16 : Constant  Value=0.4
  Constant2 : Constant  Value=0.5
  Constant28 : Constant  Value=0.8
  Constant3 : Constant  Value=5
  Constant30 : Constant  Commented=on  Value=2
  Constant4 : Constant  Value=5
  Constant7 : Constant  Commented=on
  Delay : Delay  DelayLength=1  InitialCondition=0
  Delay1 : Delay  DelayLength=1  InitialCondition=0
  Delay2 : Delay  DelayLength=1  InitialCondition=0
  Demux : Demux  Outputs=2
  Derivative : Derivative  Commented=on
  Derivative1 : Derivative
  Display2 : Display
  Display3 : Display
  From37 : From  Commented=on  GotoTag=x1
  From38 : From  Commented=on  GotoTag=x2
  Goto15 : Goto  Commented=on  GotoTag=m
  Goto16 : Goto  Commented=on  GotoTag=r
  Goto17 : Goto  Commented=on  GotoTag=d1
  Goto18 : Goto  Commented=on  GotoTag=d2
  Goto34 : Goto  Commented=on  GotoTag=d1
  Goto37 : Goto  Commented=on  GotoTag=d2
  Goto41 : Goto  Commented=on  GotoTag=xd
  Goto53 : Goto  Commented=on  GotoTag=dxd
  Goto60 : Goto  Commented=on  GotoTag=dxd
  Goto62 : Goto  Commented=on  GotoTag=ddxd
  Goto63 : Goto  Commented=on  GotoTag=xd
  Integrator3 : Integrator
  Integrator4 : Integrator
  MATLAB Function1 : MATLAB Function  TreatAsAtomicUnit=on
  MATLAB Function10 : MATLAB Function  TreatAsAtomicUnit=on
  MATLAB Function11 : MATLAB Function  TreatAsAtomicUnit=on
  MATLAB Function12 : MATLAB Function  Commented=on  TreatAsAtomicUnit=on
  MATLAB Function13 : MATLAB Function  TreatAsAtomicUnit=on
  MATLAB Function14 : MATLAB Function  TreatAsAtomicUnit=on
  MATLAB Function2 : MATLAB Function  TreatAsAtomicUnit=on
  MATLAB Function3 : MATLAB Function  TreatAsAtomicUnit=on
  MATLAB Function5 : MATLAB Function  TreatAsAtomicUnit=on
  MATLAB Function7 : MATLAB Function  Commented=on  TreatAsAtomicUnit=on
  MATLAB Function8 : MATLAB Function  TreatAsAtomicUnit=on
  MATLAB Function9 : MATLAB Function  TreatAsAtomicUnit=on
  Mux : Mux  Inputs=5
  Product1 : Product
  S-Function : S-Function  FunctionName=follower2  SFunctionDeploymentMode=off  EnableBusSupport=off
  Saturation1 : Saturate  UpperLimit=1000  LowerLimit=-1000
  Scope{,7,10,15} (4 alike) : Scope  NumInputPorts=2
  Scope{2..3,5,9,11..12,16,31..32} (9 alike) : Scope
  Scope13 : Scope  Commented=on
  Scope14 : Scope  Commented=on
  Sine Wave1 : Sin  Amplitude=0.5  Phase=pi/2  SampleTime=0
  Sine Wave2 : Sin  Amplitude=0.8*0.5  SampleTime=0
  Sine Wave4 : Sin  Commented=on  Amplitude=3  Phase=pi/2  SampleTime=0
  x1 : Outport
  x2 : Outport  Port=2
  z1 : Outport  Port=3
  z2 : Outport  Port=4
  u : Outport  Port=5
  m : Outport  Port=6
  r : Outport  Port=7
  d1 : Outport  Port=8
  d2 : Outport  Port=9
  m_u_r : Outport  Port=10
  attack_disturbance : Outport  Port=11
  IAE : Outport  Port=12
  ITAE : Outport  Port=13
  wires:
  [xd] -> Add/1, Scope/1
  Abs3/1 -> Integrator4/1
  Constant2/1 -> [beta]
  Constant4/1 -> [lada2]
  [r] -> MATLAB Function13/3(r)
  Demux/2 -> Add2/1, Scope3/1, x2/1, [x2]
  Constant/1 -> [L]
  Constant11/1 -> Goto16/1
  Constant13/1 -> Goto18/1
  MATLAB Function13/1(y) -> m_u_r/1, [m_uu_r], Scope15/2
  Demux/1 -> Add/2, x1/1, Scope/2, [x1]
  Add/1 -> z1/1, [z1], Scope5/1
  [u] -> u/1, Scope2/1, Mux/1
  Product1/1 -> Integrator3/1
  S-Function/1 -> Demux/1
  [d1] -> Mux/4
  Clock3/1 -> Product1/1
  [d2] -> MATLAB Function11/1(d2)  "d1"
  Integrator4/1 -> IAE/1, Display3/1
  Constant3/1 -> [lada1]
  [m] -> Mux/2
  Abs2/1 -> Product1/2
  Integrator3/1 -> ITAE/1, Display2/1
  Constant1/1 -> [Te]
  [r] -> MATLAB Function11/4(r)
  [z1] -> Abs2/1, Abs3/1
  Constant7/1 -> Goto15/1
  [r] -> Mux/3
  [d2] -> Mux/5
  Constant12/1 -> Goto17/1
  Mux/1 -> S-Function/1
  MATLAB Function10/1(y) -> r/1, [r], Scope12/1
  Add2/1 -> z2/1, [z2], Scope9/1
  MATLAB Function12/1(y) -> Goto34/1, Scope13/1
  Clock4/1 -> MATLAB Function10/1(u)
  Clock2/1 -> MATLAB Function9/1(t)
  MATLAB Function9/1(y) -> m/1, [m], Scope11/1
  [alph1] -> Add2/2
  [u] -> MATLAB Function11/2(u)
  [m] -> MATLAB Function11/3(m)
  MATLAB Function11/1(y) -> attack_disturbance/1, [attack_disturbance]
  [u] -> Scope15/1, MATLAB Function13/1(u)
  Sine Wave4/1 -> Scope14/1, Goto37/1
  From38/1 -> MATLAB Function12/3(x2)
  From37/1 -> MATLAB Function12/2(x1)
  Clock5/1 -> MATLAB Function12/1(t)
  [m] -> MATLAB Function13/2(m)
  Sine Wave1/1 -> d1/1, Scope31/1, [d1]
  Sine Wave2/1 -> d2/1, Scope32/1, [d2]
  MATLAB Function5/1(x1d) -> [xd]
  Constant16/1 -> MATLAB Function5/2(a)
  Constant28/1 -> MATLAB Function5/3(b)
  MATLAB Function7/3(ddx1d) -> Goto62/1
  Constant30/1 -> MATLAB Function7/2(a)
  MATLAB Function7/2(dx1d) -> Goto60/1
  In1/1 -> MATLAB Function7/3(data), MATLAB Function5/4(data), Goto41/1, Derivative/1
  Clock1/1 -> MATLAB Function5/1(t)
  Clock6/1 -> MATLAB Function7/1(t)
  Derivative/1 -> Goto53/1
  MATLAB Function5/3(ddx1d) -> [ddxd]
  MATLAB Function5/2(dx1d) -> [dxd]
  MATLAB Function7/1(x1d) -> Goto63/1
  Derivative1/1 -> MATLAB Function8/7(dalph1)
  [x2] -> MATLAB Function8/2(x2)
  [alph1] -> MATLAB Function8/6(alph1), Derivative1/1
  Saturation1/1 -> Scope16/1, [u]
  [x1] -> MATLAB Function8/1(x1)
  [x2] -> MATLAB Function1/2(x2)
  [xi_2k] -> MATLAB Function8/4(xi_2k)
  [xd] -> MATLAB Function3/4(xd)
  [u] -> MATLAB Function2/3(u)
  MATLAB Function3/1(alph1) -> [alph1]
  [alph1] -> MATLAB Function14/3(alph1)
  Delay1/1 -> [xi_2k], MATLAB Function2/4(xi_2k)
  Delay/1 -> [xi_1k], MATLAB Function1/3(xi_1k)
  MATLAB Function8/1(alph2) -> [alph2]
  Delay2/1 -> [d2_hat]
  [x2] -> MATLAB Function14/1(x2)
  [d2_hat] -> MATLAB Function8/5(d2_hat)
  [dxd] -> MATLAB Function3/5(dxd)
  MATLAB Function2/2(xi_2) -> Delay1/1
  [x1] -> MATLAB Function2/1(x1)
  MATLAB Function2/1(d2_hat) -> Delay2/1, Scope10/1
  [xd] -> MATLAB Function8/3(xd)
  [alph2] -> MATLAB Function14/4(alph2)
  [x2] -> MATLAB Function2/2(x2)
  [xi_1k] -> MATLAB Function3/2(xi_1)
  [x1] -> MATLAB Function3/1(x1)
  [d1] -> Scope7/2
  [xi_2k] -> MATLAB Function14/2(xi_2k)
  [attack_disturbance] -> Scope10/2
  [d1_hat] -> MATLAB Function3/3(d1_hat)
  MATLAB Function1/2(xi_1) -> Delay/1
  MATLAB Function14/1(u) -> Saturation1/1
  MATLAB Function1/1(d1_hat) -> Scope7/1, [d1_hat]
  [x1] -> MATLAB Function1/1(x1)

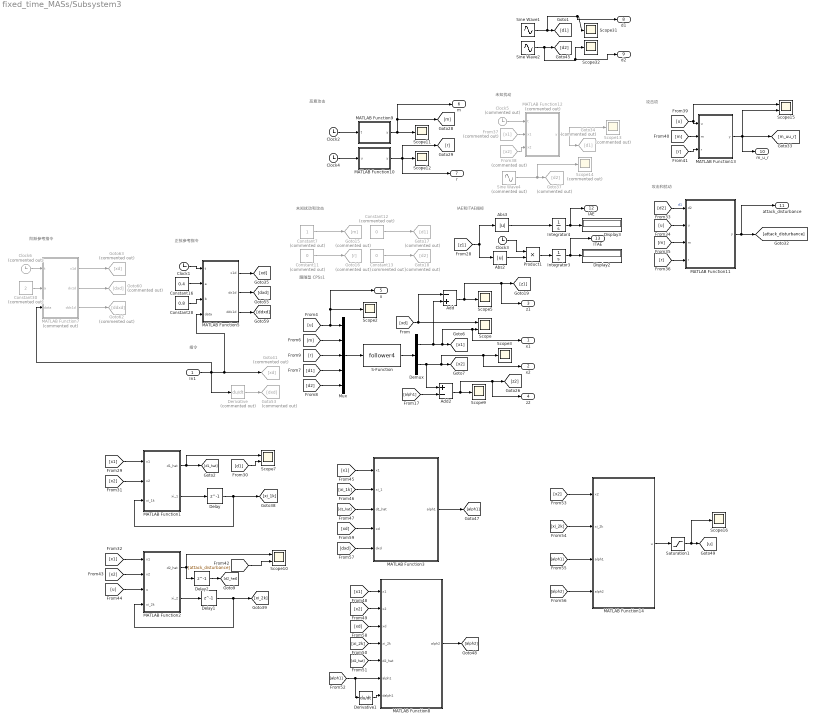
== system fixed_time_MASs/Subsystem3 ==
  note: 攻击项
  note: 攻击和扰动
  note: 未知扰动
  note: 恶意攻击
  note: IAE和ITAE指标
  note: 未知扰动和攻击
  note: 跟随型 CPSs1
  note: 正弦参考指令
  note: 阶跃参考指令
  note: 指令
  In1 : Inport
  Abs2 : Abs  SaturateOnIntegerOverflow=off
  Abs3 : Abs  SaturateOnIntegerOverflow=off
  Add : Sum  Inputs=-+
  Add2 : Sum  Inputs=+-
  Clock{1..4} (4 alike) : Clock
  Clock5 : Clock  Commented=on
  Clock6 : Clock  Commented=on
  Constant11 : Constant  Commented=on  Value=0
  Constant12 : Constant  Commented=on  Value=0
  Constant13 : Constant  Commented=on  Value=0
  Constant16 : Constant  Value=0.4
  Constant28 : Constant  Value=0.8
  Constant30 : Constant  Commented=on  Value=2
  Constant7 : Constant  Commented=on
  Delay : Delay  DelayLength=1  InitialCondition=0
  Delay1 : Delay  DelayLength=1  InitialCondition=0
  Delay2 : Delay  DelayLength=1  InitialCondition=0
  Demux : Demux  Outputs=2
  Derivative : Derivative  Commented=on
  Derivative1 : Derivative
  Display2 : Display
  Display3 : Display
  From37 : From  Commented=on  GotoTag=x1
  From38 : From  Commented=on  GotoTag=x2
  Goto15 : Goto  Commented=on  GotoTag=m
  Goto16 : Goto  Commented=on  GotoTag=r
  Goto17 : Goto  Commented=on  GotoTag=d1
  Goto18 : Goto  Commented=on  GotoTag=d2
  Goto34 : Goto  Commented=on  GotoTag=d1
  Goto37 : Goto  Commented=on  GotoTag=d2
  Goto41 : Goto  Commented=on  GotoTag=xd
  Goto53 : Goto  Commented=on  GotoTag=dxd
  Goto60 : Goto  Commented=on  GotoTag=dxd
  Goto62 : Goto  Commented=on  GotoTag=ddxd
  Goto63 : Goto  Commented=on  GotoTag=xd
  Integrator3 : Integrator
  Integrator4 : Integrator
  MATLAB Function1 : MATLAB Function  TreatAsAtomicUnit=on
  MATLAB Function10 : MATLAB Function  TreatAsAtomicUnit=on
  MATLAB Function11 : MATLAB Function  TreatAsAtomicUnit=on
  MATLAB Function12 : MATLAB Function  Commented=on  TreatAsAtomicUnit=on
  MATLAB Function13 : MATLAB Function  TreatAsAtomicUnit=on
  MATLAB Function14 : MATLAB Function  TreatAsAtomicUnit=on
  MATLAB Function2 : MATLAB Function  TreatAsAtomicUnit=on
  MATLAB Function3 : MATLAB Function  TreatAsAtomicUnit=on
  MATLAB Function5 : MATLAB Function  TreatAsAtomicUnit=on
  MATLAB Function7 : MATLAB Function  Commented=on  TreatAsAtomicUnit=on
  MATLAB Function8 : MATLAB Function  TreatAsAtomicUnit=on
  MATLAB Function9 : MATLAB Function  TreatAsAtomicUnit=on
  Mux : Mux  Inputs=5
  Product1 : Product
  S-Function : S-Function  FunctionName=follower4  SFunctionDeploymentMode=off  EnableBusSupport=off
  Saturation1 : Saturate  UpperLimit=1000  LowerLimit=-1000
  Scope{,7,10,15} (4 alike) : Scope  NumInputPorts=2
  Scope{2..3,5,9,11..12,16,31..32} (9 alike) : Scope
  Scope13 : Scope  Commented=on
  Scope14 : Scope  Commented=on
  Sine Wave1 : Sin  Phase=pi/2  SampleTime=0
  Sine Wave2 : Sin  Amplitude=0.8  SampleTime=0
  Sine Wave4 : Sin  Commented=on  Amplitude=3  Phase=pi/2  SampleTime=0
  x1 : Outport
  x2 : Outport  Port=2
  z1 : Outport  Port=3
  z2 : Outport  Port=4
  u : Outport  Port=5
  m : Outport  Port=6
  r : Outport  Port=7
  d1 : Outport  Port=8
  d2 : Outport  Port=9
  m_u_r : Outport  Port=10
  attack_disturbance : Outport  Port=11
  IAE : Outport  Port=12
  ITAE : Outport  Port=13
  wires:
  [m] -> MATLAB Function13/2(m)
  Clock5/1 -> MATLAB Function12/1(t)
  From37/1 -> MATLAB Function12/2(x1)
  From38/1 -> MATLAB Function12/3(x2)
  Sine Wave4/1 -> Goto37/1, Scope14/1
  [u] -> MATLAB Function13/1(u), Scope15/1
  MATLAB Function11/1(y) -> [attack_disturbance], attack_disturbance/1
  [m] -> MATLAB Function11/3(m)
  [u] -> MATLAB Function11/2(u)
  [alph1] -> Add2/2
  MATLAB Function9/1(y) -> Scope11/1, [m], m/1
  Clock2/1 -> MATLAB Function9/1(t)
  Clock4/1 -> MATLAB Function10/1(u)
  MATLAB Function12/1(y) -> Scope13/1, Goto34/1
  Add2/1 -> Scope9/1, [z2], z2/1
  MATLAB Function10/1(y) -> Scope12/1, [r], r/1
  Mux/1 -> S-Function/1
  Constant12/1 -> Goto17/1
  [d2] -> Mux/5
  [r] -> Mux/3
  Constant7/1 -> Goto15/1
  [z1] -> Abs3/1, Abs2/1
  [r] -> MATLAB Function11/4(r)
  Integrator3/1 -> Display2/1, ITAE/1
  Abs2/1 -> Product1/2
  [m] -> Mux/2
  Integrator4/1 -> Display3/1, IAE/1
  [d2] -> MATLAB Function11/1(d2)  "d1"
  Clock3/1 -> Product1/1
  [d1] -> Mux/4
  S-Function/1 -> Demux/1
  Product1/1 -> Integrator3/1
  [u] -> Mux/1, Scope2/1, u/1
  Add/1 -> Scope5/1, [z1], z1/1
  Demux/1 -> [x1], Scope/2, x1/1, Add/2
  MATLAB Function13/1(y) -> Scope15/2, [m_uu_r], m_u_r/1
  Constant13/1 -> Goto18/1
  Constant11/1 -> Goto16/1
  Demux/2 -> [x2], x2/1, Scope3/1, Add2/1
  [r] -> MATLAB Function13/3(r)
  Abs3/1 -> Integrator4/1
  [xd] -> Scope/1, Add/1
  Sine Wave1/1 -> d1/1, Scope31/1, [d1]
  Sine Wave2/1 -> d2/1, Scope32/1, [d2]
  MATLAB Function5/1(x1d) -> [xd]
  Constant16/1 -> MATLAB Function5/2(a)
  Constant28/1 -> MATLAB Function5/3(b)
  MATLAB Function7/3(ddx1d) -> Goto62/1
  Constant30/1 -> MATLAB Function7/2(a)
  MATLAB Function7/2(dx1d) -> Goto60/1
  In1/1 -> MATLAB Function7/3(data), MATLAB Function5/4(data), Goto41/1, Derivative/1
  Clock1/1 -> MATLAB Function5/1(t)
  Clock6/1 -> MATLAB Function7/1(t)
  Derivative/1 -> Goto53/1
  MATLAB Function5/3(ddx1d) -> [ddxd]
  MATLAB Function5/2(dx1d) -> [dxd]
  MATLAB Function7/1(x1d) -> Goto63/1
  Derivative1/1 -> MATLAB Function8/7(dalph1)
  [x2] -> MATLAB Function8/2(x2)
  [alph1] -> MATLAB Function8/6(alph1), Derivative1/1
  Saturation1/1 -> Scope16/1, [u]
  [x1] -> MATLAB Function8/1(x1)
  [x2] -> MATLAB Function1/2(x2)
  [xi_2k] -> MATLAB Function8/4(xi_2k)
  [xd] -> MATLAB Function3/4(xd)
  [u] -> MATLAB Function2/3(u)
  MATLAB Function3/1(alph1) -> [alph1]
  [alph1] -> MATLAB Function14/3(alph1)
  Delay1/1 -> [xi_2k], MATLAB Function2/4(xi_2k)
  Delay/1 -> [xi_1k], MATLAB Function1/3(xi_1k)
  MATLAB Function8/1(alph2) -> [alph2]
  Delay2/1 -> [d2_hat]
  [x2] -> MATLAB Function14/1(x2)
  [d2_hat] -> MATLAB Function8/5(d2_hat)
  [dxd] -> MATLAB Function3/5(dxd)
  MATLAB Function2/2(xi_2) -> Delay1/1
  [x1] -> MATLAB Function2/1(x1)
  MATLAB Function2/1(d2_hat) -> Delay2/1, Scope10/1
  [xd] -> MATLAB Function8/3(xd)
  [alph2] -> MATLAB Function14/4(alph2)
  [x2] -> MATLAB Function2/2(x2)
  [xi_1k] -> MATLAB Function3/2(xi_1)
  [x1] -> MATLAB Function3/1(x1)
  [d1] -> Scope7/2
  [xi_2k] -> MATLAB Function14/2(xi_2k)
  [attack_disturbance] -> Scope10/2
  [d1_hat] -> MATLAB Function3/3(d1_hat)
  MATLAB Function1/2(xi_1) -> Delay/1
  MATLAB Function14/1(u) -> Saturation1/1
  MATLAB Function1/1(d1_hat) -> Scope7/1, [d1_hat]
  [x1] -> MATLAB Function1/1(x1)

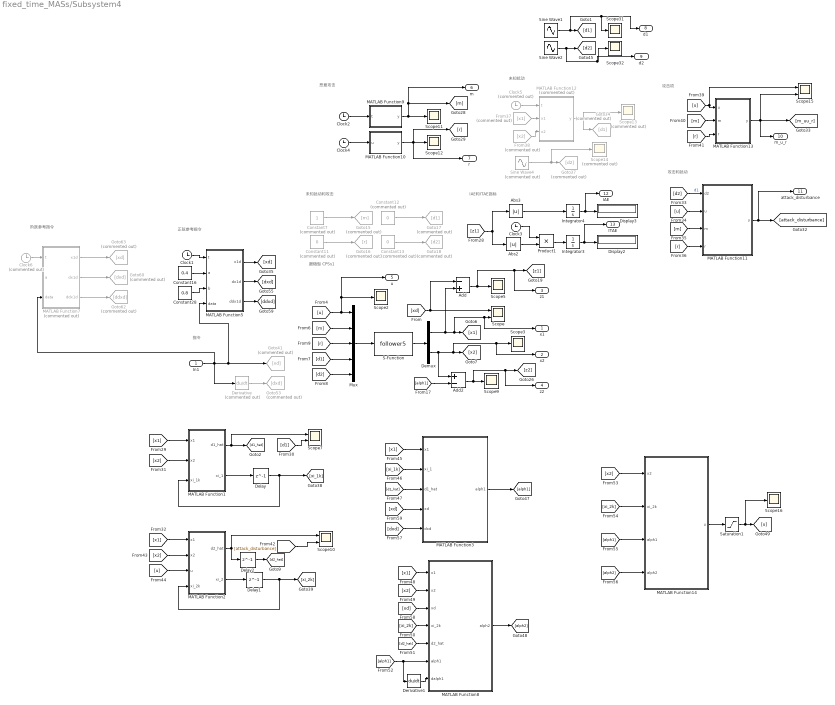
== system fixed_time_MASs/Subsystem4 ==
  note: 跟随型 CPSs1
  note: 未知扰动和攻击
  note: IAE和ITAE指标
  note: 恶意攻击
  note: 未知扰动
  note: 攻击和扰动
  note: 攻击项
  note: 正弦参考指令
  note: 阶跃参考指令
  note: 指令
  In1 : Inport
  Abs2 : Abs  SaturateOnIntegerOverflow=off
  Abs3 : Abs  SaturateOnIntegerOverflow=off
  Add : Sum  Inputs=-+
  Add2 : Sum  Inputs=+-
  Clock{1..4} (4 alike) : Clock
  Clock5 : Clock  Commented=on
  Clock6 : Clock  Commented=on
  Constant11 : Constant  Commented=on  Value=0
  Constant12 : Constant  Commented=on  Value=0
  Constant13 : Constant  Commented=on  Value=0
  Constant16 : Constant  Value=0.4
  Constant28 : Constant  Value=0.8
  Constant7 : Constant  Commented=on
  Delay : Delay  DelayLength=1  InitialCondition=0
  Delay1 : Delay  DelayLength=1  InitialCondition=0
  Delay2 : Delay  DelayLength=1  InitialCondition=0
  Demux : Demux  Outputs=2
  Derivative : Derivative  Commented=on
  Derivative1 : Derivative
  Display2 : Display
  Display3 : Display
  From37 : From  Commented=on  GotoTag=x1
  From38 : From  Commented=on  GotoTag=x2
  Goto15 : Goto  Commented=on  GotoTag=m
  Goto16 : Goto  Commented=on  GotoTag=r
  Goto17 : Goto  Commented=on  GotoTag=d1
  Goto18 : Goto  Commented=on  GotoTag=d2
  Goto34 : Goto  Commented=on  GotoTag=d1
  Goto37 : Goto  Commented=on  GotoTag=d2
  Goto41 : Goto  Commented=on  GotoTag=xd
  Goto53 : Goto  Commented=on  GotoTag=dxd
  Goto60 : Goto  Commented=on  GotoTag=dxd
  Goto62 : Goto  Commented=on  GotoTag=ddxd
  Goto63 : Goto  Commented=on  GotoTag=xd
  Integrator3 : Integrator
  Integrator4 : Integrator
  MATLAB Function1 : MATLAB Function  TreatAsAtomicUnit=on
  MATLAB Function10 : MATLAB Function  TreatAsAtomicUnit=on
  MATLAB Function11 : MATLAB Function  TreatAsAtomicUnit=on
  MATLAB Function12 : MATLAB Function  Commented=on  TreatAsAtomicUnit=on
  MATLAB Function13 : MATLAB Function  TreatAsAtomicUnit=on
  MATLAB Function14 : MATLAB Function  TreatAsAtomicUnit=on
  MATLAB Function2 : MATLAB Function  TreatAsAtomicUnit=on
  MATLAB Function3 : MATLAB Function  TreatAsAtomicUnit=on
  MATLAB Function5 : MATLAB Function  TreatAsAtomicUnit=on
  MATLAB Function7 : MATLAB Function  Commented=on  TreatAsAtomicUnit=on
  MATLAB Function8 : MATLAB Function  TreatAsAtomicUnit=on
  MATLAB Function9 : MATLAB Function  TreatAsAtomicUnit=on
  Mux : Mux  Inputs=5
  Product1 : Product
  S-Function : S-Function  FunctionName=follower5  SFunctionDeploymentMode=off  EnableBusSupport=off
  Saturation1 : Saturate  UpperLimit=1000  LowerLimit=-1000
  Scope{,7,10,15} (4 alike) : Scope  NumInputPorts=2
  Scope{2..3,5,9,11..12,16,31..32} (9 alike) : Scope
  Scope13 : Scope  Commented=on
  Scope14 : Scope  Commented=on
  Sine Wave1 : Sin  Amplitude=1.2  Phase=pi/2  SampleTime=0
  Sine Wave2 : Sin  Amplitude=0.8*1.2  SampleTime=0
  Sine Wave4 : Sin  Commented=on  Amplitude=3  Phase=pi/2  SampleTime=0
  x1 : Outport
  x2 : Outport  Port=2
  z1 : Outport  Port=3
  z2 : Outport  Port=4
  u : Outport  Port=5
  m : Outport  Port=6
  r : Outport  Port=7
  d1 : Outport  Port=8
  d2 : Outport  Port=9
  m_u_r : Outport  Port=10
  attack_disturbance : Outport  Port=11
  IAE : Outport  Port=12
  ITAE : Outport  Port=13
  wires:
  [xd] -> Add/1, Scope/1
  Abs3/1 -> Integrator4/1
  [r] -> MATLAB Function13/3(r)
  Demux/2 -> Add2/1, Scope3/1, x2/1, [x2]
  Constant11/1 -> Goto16/1
  Constant13/1 -> Goto18/1
  MATLAB Function13/1(y) -> m_u_r/1, [m_uu_r], Scope15/2
  Demux/1 -> Add/2, x1/1, Scope/2, [x1]
  Add/1 -> z1/1, [z1], Scope5/1
  [u] -> u/1, Scope2/1, Mux/1
  Product1/1 -> Integrator3/1
  S-Function/1 -> Demux/1
  [d1] -> Mux/4
  Clock3/1 -> Product1/1
  [d2] -> MATLAB Function11/1(d2)  "d1"
  Integrator4/1 -> IAE/1, Display3/1
  [m] -> Mux/2
  Abs2/1 -> Product1/2
  Integrator3/1 -> ITAE/1, Display2/1
  [r] -> MATLAB Function11/4(r)
  [z1] -> Abs2/1, Abs3/1
  Constant7/1 -> Goto15/1
  [r] -> Mux/3
  [d2] -> Mux/5
  Constant12/1 -> Goto17/1
  Mux/1 -> S-Function/1
  MATLAB Function10/1(y) -> r/1, [r], Scope12/1
  Add2/1 -> z2/1, [z2], Scope9/1
  MATLAB Function12/1(y) -> Goto34/1, Scope13/1
  Clock4/1 -> MATLAB Function10/1(u)
  Clock2/1 -> MATLAB Function9/1(t)
  MATLAB Function9/1(y) -> m/1, [m], Scope11/1
  [alph1] -> Add2/2
  [u] -> MATLAB Function11/2(u)
  [m] -> MATLAB Function11/3(m)
  MATLAB Function11/1(y) -> attack_disturbance/1, [attack_disturbance]
  [u] -> Scope15/1, MATLAB Function13/1(u)
  Sine Wave4/1 -> Scope14/1, Goto37/1
  From38/1 -> MATLAB Function12/3(x2)
  From37/1 -> MATLAB Function12/2(x1)
  Clock5/1 -> MATLAB Function12/1(t)
  [m] -> MATLAB Function13/2(m)
  Sine Wave1/1 -> d1/1, Scope31/1, [d1]
  Sine Wave2/1 -> d2/1, Scope32/1, [d2]
  MATLAB Function5/1(x1d) -> [xd]
  Constant16/1 -> MATLAB Function5/2(a)
  Constant28/1 -> MATLAB Function5/3(b)
  MATLAB Function7/1(x1d) -> Goto63/1
  MATLAB Function7/3(ddx1d) -> Goto62/1
  ? -> MATLAB Function7/2(a)
  MATLAB Function7/2(dx1d) -> Goto60/1
  In1/1 -> MATLAB Function7/3(data), MATLAB Function5/4(data), Goto41/1, Derivative/1
  Clock1/1 -> MATLAB Function5/1(t)
  Clock6/1 -> MATLAB Function7/1(t)
  Derivative/1 -> Goto53/1
  MATLAB Function5/3(ddx1d) -> [ddxd]
  MATLAB Function5/2(dx1d) -> [dxd]
  Derivative1/1 -> MATLAB Function8/7(dalph1)
  [x2] -> MATLAB Function8/2(x2)
  [alph1] -> MATLAB Function8/6(alph1), Derivative1/1
  Saturation1/1 -> Scope16/1, [u]
  [x1] -> MATLAB Function8/1(x1)
  [x2] -> MATLAB Function1/2(x2)
  [xi_2k] -> MATLAB Function8/4(xi_2k)
  [xd] -> MATLAB Function3/4(xd)
  [u] -> MATLAB Function2/3(u)
  MATLAB Function3/1(alph1) -> [alph1]
  [alph1] -> MATLAB Function14/3(alph1)
  Delay1/1 -> [xi_2k], MATLAB Function2/4(xi_2k)
  Delay/1 -> [xi_1k], MATLAB Function1/3(xi_1k)
  MATLAB Function8/1(alph2) -> [alph2]
  Delay2/1 -> [d2_hat]
  [x2] -> MATLAB Function14/1(x2)
  [d2_hat] -> MATLAB Function8/5(d2_hat)
  [dxd] -> MATLAB Function3/5(dxd)
  MATLAB Function2/2(xi_2) -> Delay1/1
  [x1] -> MATLAB Function2/1(x1)
  MATLAB Function2/1(d2_hat) -> Delay2/1, Scope10/1
  [xd] -> MATLAB Function8/3(xd)
  [alph2] -> MATLAB Function14/4(alph2)
  [x2] -> MATLAB Function2/2(x2)
  [xi_1k] -> MATLAB Function3/2(xi_1)
  [x1] -> MATLAB Function3/1(x1)
  [d1] -> Scope7/2
  [xi_2k] -> MATLAB Function14/2(xi_2k)
  [attack_disturbance] -> Scope10/2
  [d1_hat] -> MATLAB Function3/3(d1_hat)
  MATLAB Function1/2(xi_1) -> Delay/1
  MATLAB Function14/1(u) -> Saturation1/1
  MATLAB Function1/1(d1_hat) -> Scope7/1, [d1_hat]
  [x1] -> MATLAB Function1/1(x1)

== matlab function fixed_time_MASs/Subsystem/MATLAB Function13 ==
  data: u input; y output; m input; r input
function y = fcn(u, m, r)
y=m*u+r;

== matlab function fixed_time_MASs/Subsystem/MATLAB Function7 ==
  data: t input; x1d output; dx1d output; ddx1d output; a input; data input
function [x1d, dx1d, ddx1d] = fcn(t,a, data)
% if t<5
%     x1d = 0;
% else
%     x1d = a;
% end
x1d = data;
dx1d = 0;
ddx1d = 0;

== matlab function fixed_time_MASs/Subsystem/MATLAB Function1 ==
  data: d1_hat output; x1 input; x2 input; xi_1 output; xi_1k input
function [d1_hat, xi_1] = fcn(x1, x2, xi_1k)

f1 = 0.8*x1*sin(x1*x1);
fi0 = 1; fi1 = 5; fi2 = 5;
% a1 = 123; q1 = 101; 
% h1 = 91; n1 = 101;
a1 = 7; q1 = 10; 
h1 = 13; n1 = 10;
Ts = 0.0001;

xi_1 = xi_1k+Ts*(x2+f1-fi0*(xi_1k-x1)-fi1*(abs(xi_1k-x1)^(a1/q1))*sign(xi_1k-x1)-fi2*(abs(xi_1k-x1)^(h1/n1))*sign(xi_1k-x1));
d1_hat = -fi0*(xi_1k-x1)-fi1*(abs(xi_1k-x1)^(a1/q1))*sign(xi_1k-x1)-fi2*(abs(xi_1k-x1)^(h1/n1))*sign(xi_1k-x1);
